simulink model "orion_casestudy_8"  (R2023a)
settings: Solver=VariableStepAuto  StartTime=0.0  StopTime=30  RelTol=1e-3
InitFcn:
  | RandStream.setGlobalStream(RandStream('mt19937ar','seed',sum(100*clock)));
undefined symbols (not defined in the file or in its folder): m, n
(part 2 of 3)

== stateflow chart orion_casestudy_8/Slave3 ==
  settings: updateMethod=CONTINUOUS
  state Connected
    entry:
    connStatus=2;
    state KeepAliveSendTimeout [parallel]
      settings: executionOrder=1
      state KeepAliveSend
      (default) -> KeepAliveSend
      KeepAliveSend -> KeepAliveSend [order 1] : after(delay_array(i)*5,msec)
          |  {OrionKeepAliveOut.data=0;
          | send(OrionKeepAliveOut);i = i + 1;}
      KeepAliveSend -> KeepAliveSend [order 2] : SendDataIn
          | {OrionAppDataOut.data=0;
          | send(OrionAppDataOut);}
    state KeepAliveRecieveTimeout [parallel]
      settings: executionOrder=2
      state KeepAlineRec
      (default) -> KeepAlineRec
      KeepAlineRec -> KeepAlineRec [order 2] : OrionKeepAliveIn
      KeepAlineRec -> KeepAlineRec [order 3] : OrionAppDataIn
  state Closed
    entry:
    connStatus=0;
  state Connecting
    entry:
    connStatus=1;
  Connected -> (junction 6) [order 2] : OrionConnRespIn
  Connected -> (junction 6) [order 3] : OrionConnReqIn
  (default) -> Closed : {i=1;}
  (junction 6) -> Closed
  Connected -> (junction 6) [order 1] : OrionConnConfIn
  KeepAlineRec -> Closed [order 1] : after(delay_array(i)*5,msec)
      | {i = i + 1;}
  Connecting -> (junction 36) [order 6] : OrionAppDataIn
  Connecting -> (junction 36) [order 5] : OrionConnReqIn
  (junction 36) -> Closed
  Connecting -> (junction 36) [order 4] : OrionConnRespIn
  Connecting -> (junction 36) [order 3] : OrionKeepAliveIn
  Closed -> Connecting : OrionConnReqIn
      | {OrionConnRespOut.data=0;
      | send(OrionConnRespOut);}
  Connecting -> Closed [order 1] : after(delay_array(i)*5,msec)
      | {i = i + 1;}
  Connecting -> Connected [order 2] : OrionConnConfIn{OrionConnConfOut.data=0;send(OrionConnConfOut);}
  data: OrionKeepAliveIn input; OrionConnConfOut output; OrionConnRespOut output; OrionKeepAliveOut output; OrionAppDataOut output; OrionAppDataIn input; OrionConnRespIn input; OrionConnReqIn input; OrionConnReqOut output size=1; connStatus output; SendDataIn local; OrionConnConfIn input; delay_array input; i local

== stateflow chart orion_casestudy_8/DelaySwitch41 ==
  state Operation
  state Sending
  (default) -> Operation : {i=0;}
  (junction 7) -> Operation [order 2]
  Sending -> Operation : after(delay_array(i),msec)
      | {receive(inMsg);outMsg.data=0;send(outMsg);}
  Operation -> (junction 7) : inMsg{i = i + 1;}
  (junction 7) -> Sending [order 1] : [switch_array(i)==0]
  data: switch_array input; delay_array input; outMsg output; inMsg input; i local

== stateflow chart orion_casestudy_8/DelaySwitch42 ==
  state Operation
  state Sending
  (default) -> Operation : {i=0;}
  (junction 7) -> Operation [order 2]
  Sending -> Operation : after(delay_array(i),msec)
      | {receive(inMsg);outMsg.data=0;send(outMsg);}
  Operation -> (junction 7) : inMsg{i = i + 1;}
  (junction 7) -> Sending [order 1] : [switch_array(i)==0]
  data: switch_array input; delay_array input; outMsg output; inMsg input; i local

== stateflow chart orion_casestudy_8/DelaySwitch43 ==
  state Operation
  state Sending
  (default) -> Operation : {i=0;}
  (junction 7) -> Operation [order 2]
  Sending -> Operation : after(delay_array(i),msec)
      | {receive(inMsg);outMsg.data=0;send(outMsg);}
  Operation -> (junction 7) : inMsg{i = i + 1;}
  (junction 7) -> Sending [order 1] : [switch_array(i)==0]
  data: switch_array input; delay_array input; outMsg output; inMsg input; i local

== stateflow chart orion_casestudy_8/DelaySwitch44 ==
  state Operation
  state Sending
  (default) -> Operation : {i=0;}
  (junction 7) -> Operation [order 2]
  Sending -> Operation : after(delay_array(i),msec)
      | {receive(inMsg);outMsg.data=0;send(outMsg);}
  Operation -> (junction 7) : inMsg{i = i + 1;}
  (junction 7) -> Sending [order 1] : [switch_array(i)==0]
  data: switch_array input; delay_array input; outMsg output; inMsg input; i local

== stateflow chart orion_casestudy_8/DelaySwitch45 ==
  state Operation
  state Sending
  (default) -> Operation : {i=0;}
  (junction 7) -> Operation [order 2]
  Sending -> Operation : after(delay_array(i),msec)
      | {receive(inMsg);outMsg.data=0;send(outMsg);}
  Operation -> (junction 7) : inMsg{i = i + 1;}
  (junction 7) -> Sending [order 1] : [switch_array(i)==0]
  data: switch_array input; delay_array input; outMsg output; inMsg input; i local

== stateflow chart orion_casestudy_8/DelaySwitch46 ==
  state Operation
  state Sending
  (default) -> Operation : {i=0;}
  (junction 7) -> Operation [order 2]
  Sending -> Operation : after(delay_array(i),msec)
      | {receive(inMsg);outMsg.data=0;send(outMsg);}
  Operation -> (junction 7) : inMsg{i = i + 1;}
  (junction 7) -> Sending [order 1] : [switch_array(i)==0]
  data: switch_array input; delay_array input; outMsg output; inMsg input; i local

== stateflow chart orion_casestudy_8/DelaySwitch47 ==
  state Operation
  state Sending
  (default) -> Operation : {i=0;}
  (junction 7) -> Operation [order 2]
  Sending -> Operation : after(delay_array(i),msec)
      | {receive(inMsg);outMsg.data=0;send(outMsg);}
  Operation -> (junction 7) : inMsg{i = i + 1;}
  (junction 7) -> Sending [order 1] : [switch_array(i)==0]
  data: switch_array input; delay_array input; outMsg output; inMsg input; i local

== stateflow chart orion_casestudy_8/DelaySwitch48 ==
  state Operation
  state Sending
  (default) -> Operation : {i=0;}
  (junction 7) -> Operation [order 2]
  Sending -> Operation : after(delay_array(i),msec)
      | {receive(inMsg);outMsg.data=0;send(outMsg);}
  Operation -> (junction 7) : inMsg{i = i + 1;}
  (junction 7) -> Sending [order 1] : [switch_array(i)==0]
  data: switch_array input; delay_array input; outMsg output; inMsg input; i local

== stateflow chart orion_casestudy_8/DelaySwitch49 ==
  state Operation
  state Sending
  (default) -> Operation : {i=0;}
  (junction 7) -> Operation [order 2]
  Sending -> Operation : after(delay_array(i),msec)
      | {receive(inMsg);outMsg.data=0;send(outMsg);}
  Operation -> (junction 7) : inMsg{i = i + 1;}
  (junction 7) -> Sending [order 1] : [switch_array(i)==0]
  data: switch_array input; delay_array input; outMsg output; inMsg input; i local

== stateflow chart orion_casestudy_8/DelaySwitch50 ==
  state Operation
  state Sending
  (default) -> Operation : {i=0;}
  (junction 7) -> Operation [order 2]
  Sending -> Operation : after(delay_array(i),msec)
      | {receive(inMsg);outMsg.data=0;send(outMsg);}
  Operation -> (junction 7) : inMsg{i = i + 1;}
  (junction 7) -> Sending [order 1] : [switch_array(i)==0]
  data: switch_array input; delay_array input; outMsg output; inMsg input; i local

== stateflow chart orion_casestudy_8/DelaySwitch51 ==
  state Operation
  state Sending
  (default) -> Operation : {i=0;}
  (junction 7) -> Operation [order 2]
  Sending -> Operation : after(delay_array(i),msec)
      | {receive(inMsg);outMsg.data=0;send(outMsg);}
  Operation -> (junction 7) : inMsg{i = i + 1;}
  (junction 7) -> Sending [order 1] : [switch_array(i)==0]
  data: switch_array input; delay_array input; outMsg output; inMsg input; i local

== stateflow chart orion_casestudy_8/DelaySwitch52 ==
  state Operation
  state Sending
  (default) -> Operation : {i=0;}
  (junction 7) -> Operation [order 2]
  Sending -> Operation : after(delay_array(i),msec)
      | {receive(inMsg);outMsg.data=0;send(outMsg);}
  Operation -> (junction 7) : inMsg{i = i + 1;}
  (junction 7) -> Sending [order 1] : [switch_array(i)==0]
  data: switch_array input; delay_array input; outMsg output; inMsg input; i local

== stateflow chart orion_casestudy_8/DelaySwitch53 ==
  state Operation
  state Sending
  (default) -> Operation : {i=0;}
  (junction 7) -> Operation [order 2]
  Sending -> Operation : after(delay_array(i),msec)
      | {receive(inMsg);outMsg.data=0;send(outMsg);}
  Operation -> (junction 7) : inMsg{i = i + 1;}
  (junction 7) -> Sending [order 1] : [switch_array(i)==0]
  data: switch_array input; delay_array input; outMsg output; inMsg input; i local

== stateflow chart orion_casestudy_8/DelaySwitch54 ==
  state Operation
  state Sending
  (default) -> Operation : {i=0;}
  (junction 7) -> Operation [order 2]
  Sending -> Operation : after(delay_array(i),msec)
      | {receive(inMsg);outMsg.data=0;send(outMsg);}
  Operation -> (junction 7) : inMsg{i = i + 1;}
  (junction 7) -> Sending [order 1] : [switch_array(i)==0]
  data: switch_array input; delay_array input; outMsg output; inMsg input; i local

== stateflow chart orion_casestudy_8/DelaySwitch55 ==
  state Operation
  state Sending
  (default) -> Operation : {i=0;}
  (junction 7) -> Operation [order 2]
  Sending -> Operation : after(delay_array(i),msec)
      | {receive(inMsg);outMsg.data=0;send(outMsg);}
  Operation -> (junction 7) : inMsg{i = i + 1;}
  (junction 7) -> Sending [order 1] : [switch_array(i)==0]
  data: switch_array input; delay_array input; outMsg output; inMsg input; i local

== stateflow chart orion_casestudy_8/DelaySwitch56 ==
  state Operation
  state Sending
  (default) -> Operation : {i=0;}
  (junction 7) -> Operation [order 2]
  Sending -> Operation : after(delay_array(i),msec)
      | {receive(inMsg);outMsg.data=0;send(outMsg);}
  Operation -> (junction 7) : inMsg{i = i + 1;}
  (junction 7) -> Sending [order 1] : [switch_array(i)==0]
  data: switch_array input; delay_array input; outMsg output; inMsg input; i local

== stateflow chart orion_casestudy_8/DelaySwitch57 ==
  state Operation
  state Sending
  (default) -> Operation : {i=0;}
  (junction 7) -> Operation [order 2]
  Sending -> Operation : after(delay_array(i),msec)
      | {receive(inMsg);outMsg.data=0;send(outMsg);}
  Operation -> (junction 7) : inMsg{i = i + 1;}
  (junction 7) -> Sending [order 1] : [switch_array(i)==0]
  data: switch_array input; delay_array input; outMsg output; inMsg input; i local

== stateflow chart orion_casestudy_8/DelaySwitch58 ==
  state Operation
  state Sending
  (default) -> Operation : {i=0;}
  (junction 7) -> Operation [order 2]
  Sending -> Operation : after(delay_array(i),msec)
      | {receive(inMsg);outMsg.data=0;send(outMsg);}
  Operation -> (junction 7) : inMsg{i = i + 1;}
  (junction 7) -> Sending [order 1] : [switch_array(i)==0]
  data: switch_array input; delay_array input; outMsg output; inMsg input; i local

== stateflow chart orion_casestudy_8/DelaySwitch59 ==
  state Operation
  state Sending
  (default) -> Operation : {i=0;}
  (junction 7) -> Operation [order 2]
  Sending -> Operation : after(delay_array(i),msec)
      | {receive(inMsg);outMsg.data=0;send(outMsg);}
  Operation -> (junction 7) : inMsg{i = i + 1;}
  (junction 7) -> Sending [order 1] : [switch_array(i)==0]
  data: switch_array input; delay_array input; outMsg output; inMsg input; i local

== stateflow chart orion_casestudy_8/DelaySwitch60 ==
  state Operation
  state Sending
  (default) -> Operation : {i=0;}
  (junction 7) -> Operation [order 2]
  Sending -> Operation : after(delay_array(i),msec)
      | {receive(inMsg);outMsg.data=0;send(outMsg);}
  Operation -> (junction 7) : inMsg{i = i + 1;}
  (junction 7) -> Sending [order 1] : [switch_array(i)==0]
  data: switch_array input; delay_array input; outMsg output; inMsg input; i local

== stateflow chart orion_casestudy_8/DelaySwitch61 ==
  state Operation
  state Sending
  (default) -> Operation : {i=0;}
  (junction 7) -> Operation [order 2]
  Sending -> Operation : after(delay_array(i),msec)
      | {receive(inMsg);outMsg.data=0;send(outMsg);}
  Operation -> (junction 7) : inMsg{i = i + 1;}
  (junction 7) -> Sending [order 1] : [switch_array(i)==0]
  data: switch_array input; delay_array input; outMsg output; inMsg input; i local

== stateflow chart orion_casestudy_8/DelaySwitch62 ==
  state Operation
  state Sending
  (default) -> Operation : {i=0;}
  (junction 7) -> Operation [order 2]
  Sending -> Operation : after(delay_array(i),msec)
      | {receive(inMsg);outMsg.data=0;send(outMsg);}
  Operation -> (junction 7) : inMsg{i = i + 1;}
  (junction 7) -> Sending [order 1] : [switch_array(i)==0]
  data: switch_array input; delay_array input; outMsg output; inMsg input; i local

== stateflow chart orion_casestudy_8/DelaySwitch63 ==
  state Operation
  state Sending
  (default) -> Operation : {i=0;}
  (junction 7) -> Operation [order 2]
  Sending -> Operation : after(delay_array(i),msec)
      | {receive(inMsg);outMsg.data=0;send(outMsg);}
  Operation -> (junction 7) : inMsg{i = i + 1;}
  (junction 7) -> Sending [order 1] : [switch_array(i)==0]
  data: switch_array input; delay_array input; outMsg output; inMsg input; i local

== stateflow chart orion_casestudy_8/DelaySwitch3 ==
  state Operation
  state Sending
  (default) -> Operation : {i=0;}
  (junction 7) -> Operation [order 2]
  Sending -> Operation : after(delay_array(i),msec)
      | {receive(inMsg);outMsg.data=0;send(outMsg);}
  Operation -> (junction 7) : inMsg{i = i + 1;}
  (junction 7) -> Sending [order 1] : [switch_array(i)==0]
  data: switch_array input; delay_array input; outMsg output; inMsg input; i local

== stateflow chart orion_casestudy_8/DelaySwitch64 ==
  state Operation
  state Sending
  (default) -> Operation : {i=0;}
  (junction 7) -> Operation [order 2]
  Sending -> Operation : after(delay_array(i),msec)
      | {receive(inMsg);outMsg.data=0;send(outMsg);}
  Operation -> (junction 7) : inMsg{i = i + 1;}
  (junction 7) -> Sending [order 1] : [switch_array(i)==0]
  data: switch_array input; delay_array input; outMsg output; inMsg input; i local

== stateflow chart orion_casestudy_8/DelaySwitch65 ==
  state Operation
  state Sending
  (default) -> Operation : {i=0;}
  (junction 7) -> Operation [order 2]
  Sending -> Operation : after(delay_array(i),msec)
      | {receive(inMsg);outMsg.data=0;send(outMsg);}
  Operation -> (junction 7) : inMsg{i = i + 1;}
  (junction 7) -> Sending [order 1] : [switch_array(i)==0]
  data: switch_array input; delay_array input; outMsg output; inMsg input; i local

== stateflow chart orion_casestudy_8/DelaySwitch66 ==
  state Operation
  state Sending
  (default) -> Operation : {i=0;}
  (junction 7) -> Operation [order 2]
  Sending -> Operation : after(delay_array(i),msec)
      | {receive(inMsg);outMsg.data=0;send(outMsg);}
  Operation -> (junction 7) : inMsg{i = i + 1;}
  (junction 7) -> Sending [order 1] : [switch_array(i)==0]
  data: switch_array input; delay_array input; outMsg output; inMsg input; i local

== stateflow chart orion_casestudy_8/DelaySwitch67 ==
  state Operation
  state Sending
  (default) -> Operation : {i=0;}
  (junction 7) -> Operation [order 2]
  Sending -> Operation : after(delay_array(i),msec)
      | {receive(inMsg);outMsg.data=0;send(outMsg);}
  Operation -> (junction 7) : inMsg{i = i + 1;}
  (junction 7) -> Sending [order 1] : [switch_array(i)==0]
  data: switch_array input; delay_array input; outMsg output; inMsg input; i local

== stateflow chart orion_casestudy_8/DelaySwitch68 ==
  state Operation
  state Sending
  (default) -> Operation : {i=0;}
  (junction 7) -> Operation [order 2]
  Sending -> Operation : after(delay_array(i),msec)
      | {receive(inMsg);outMsg.data=0;send(outMsg);}
  Operation -> (junction 7) : inMsg{i = i + 1;}
  (junction 7) -> Sending [order 1] : [switch_array(i)==0]
  data: switch_array input; delay_array input; outMsg output; inMsg input; i local

== stateflow chart orion_casestudy_8/DelaySwitch69 ==
  state Operation
  state Sending
  (default) -> Operation : {i=0;}
  (junction 7) -> Operation [order 2]
  Sending -> Operation : after(delay_array(i),msec)
      | {receive(inMsg);outMsg.data=0;send(outMsg);}
  Operation -> (junction 7) : inMsg{i = i + 1;}
  (junction 7) -> Sending [order 1] : [switch_array(i)==0]
  data: switch_array input; delay_array input; outMsg output; inMsg input; i local

== stateflow chart orion_casestudy_8/DelaySwitch70 ==
  state Operation
  state Sending
  (default) -> Operation : {i=0;}
  (junction 7) -> Operation [order 2]
  Sending -> Operation : after(delay_array(i),msec)
      | {receive(inMsg);outMsg.data=0;send(outMsg);}
  Operation -> (junction 7) : inMsg{i = i + 1;}
  (junction 7) -> Sending [order 1] : [switch_array(i)==0]
  data: switch_array input; delay_array input; outMsg output; inMsg input; i local

== stateflow chart orion_casestudy_8/DelaySwitch71 ==
  state Operation
  state Sending
  (default) -> Operation : {i=0;}
  (junction 7) -> Operation [order 2]
  Sending -> Operation : after(delay_array(i),msec)
      | {receive(inMsg);outMsg.data=0;send(outMsg);}
  Operation -> (junction 7) : inMsg{i = i + 1;}
  (junction 7) -> Sending [order 1] : [switch_array(i)==0]
  data: switch_array input; delay_array input; outMsg output; inMsg input; i local

== stateflow chart orion_casestudy_8/DelaySwitch72 ==
  state Operation
  state Sending
  (default) -> Operation : {i=0;}
  (junction 7) -> Operation [order 2]
  Sending -> Operation : after(delay_array(i),msec)
      | {receive(inMsg);outMsg.data=0;send(outMsg);}
  Operation -> (junction 7) : inMsg{i = i + 1;}
  (junction 7) -> Sending [order 1] : [switch_array(i)==0]
  data: switch_array input; delay_array input; outMsg output; inMsg input; i local

== stateflow chart orion_casestudy_8/DelaySwitch73 ==
  state Operation
  state Sending
  (default) -> Operation : {i=0;}
  (junction 7) -> Operation [order 2]
  Sending -> Operation : after(delay_array(i),msec)
      | {receive(inMsg);outMsg.data=0;send(outMsg);}
  Operation -> (junction 7) : inMsg{i = i + 1;}
  (junction 7) -> Sending [order 1] : [switch_array(i)==0]
  data: switch_array input; delay_array input; outMsg output; inMsg input; i local

== stateflow chart orion_casestudy_8/DelaySwitch4 ==
  state Operation
  state Sending
  (default) -> Operation : {i=0;}
  (junction 7) -> Operation [order 2]
  Sending -> Operation : after(delay_array(i),msec)
      | {receive(inMsg);outMsg.data=0;send(outMsg);}
  Operation -> (junction 7) : inMsg{i = i + 1;}
  (junction 7) -> Sending [order 1] : [switch_array(i)==0]
  data: switch_array input; delay_array input; outMsg output; inMsg input; i local

== stateflow chart orion_casestudy_8/DelaySwitch74 ==
  state Operation
  state Sending
  (default) -> Operation : {i=0;}
  (junction 7) -> Operation [order 2]
  Sending -> Operation : after(delay_array(i),msec)
      | {receive(inMsg);outMsg.data=0;send(outMsg);}
  Operation -> (junction 7) : inMsg{i = i + 1;}
  (junction 7) -> Sending [order 1] : [switch_array(i)==0]
  data: switch_array input; delay_array input; outMsg output; inMsg input; i local

== stateflow chart orion_casestudy_8/DelaySwitch75 ==
  state Operation
  state Sending
  (default) -> Operation : {i=0;}
  (junction 7) -> Operation [order 2]
  Sending -> Operation : after(delay_array(i),msec)
      | {receive(inMsg);outMsg.data=0;send(outMsg);}
  Operation -> (junction 7) : inMsg{i = i + 1;}
  (junction 7) -> Sending [order 1] : [switch_array(i)==0]
  data: switch_array input; delay_array input; outMsg output; inMsg input; i local

== stateflow chart orion_casestudy_8/DelaySwitch76 ==
  state Operation
  state Sending
  (default) -> Operation : {i=0;}
  (junction 7) -> Operation [order 2]
  Sending -> Operation : after(delay_array(i),msec)
      | {receive(inMsg);outMsg.data=0;send(outMsg);}
  Operation -> (junction 7) : inMsg{i = i + 1;}
  (junction 7) -> Sending [order 1] : [switch_array(i)==0]
  data: switch_array input; delay_array input; outMsg output; inMsg input; i local

== stateflow chart orion_casestudy_8/DelaySwitch77 ==
  state Operation
  state Sending
  (default) -> Operation : {i=0;}
  (junction 7) -> Operation [order 2]
  Sending -> Operation : after(delay_array(i),msec)
      | {receive(inMsg);outMsg.data=0;send(outMsg);}
  Operation -> (junction 7) : inMsg{i = i + 1;}
  (junction 7) -> Sending [order 1] : [switch_array(i)==0]
  data: switch_array input; delay_array input; outMsg output; inMsg input; i local

== stateflow chart orion_casestudy_8/DelaySwitch78 ==
  state Operation
  state Sending
  (default) -> Operation : {i=0;}
  (junction 7) -> Operation [order 2]
  Sending -> Operation : after(delay_array(i),msec)
      | {receive(inMsg);outMsg.data=0;send(outMsg);}
  Operation -> (junction 7) : inMsg{i = i + 1;}
  (junction 7) -> Sending [order 1] : [switch_array(i)==0]
  data: switch_array input; delay_array input; outMsg output; inMsg input; i local

== stateflow chart orion_casestudy_8/DelaySwitch79 ==
  state Operation
  state Sending
  (default) -> Operation : {i=0;}
  (junction 7) -> Operation [order 2]
  Sending -> Operation : after(delay_array(i),msec)
      | {receive(inMsg);outMsg.data=0;send(outMsg);}
  Operation -> (junction 7) : inMsg{i = i + 1;}
  (junction 7) -> Sending [order 1] : [switch_array(i)==0]
  data: switch_array input; delay_array input; outMsg output; inMsg input; i local

== stateflow chart orion_casestudy_8/DelaySwitch80 ==
  state Operation
  state Sending
  (default) -> Operation : {i=0;}
  (junction 7) -> Operation [order 2]
  Sending -> Operation : after(delay_array(i),msec)
      | {receive(inMsg);outMsg.data=0;send(outMsg);}
  Operation -> (junction 7) : inMsg{i = i + 1;}
  (junction 7) -> Sending [order 1] : [switch_array(i)==0]
  data: switch_array input; delay_array input; outMsg output; inMsg input; i local

== stateflow chart orion_casestudy_8/Master4 ==
  settings: updateMethod=CONTINUOUS
  state Connected
    entry:
    connStatus=2;
    state KeepAliveSendTimeout [parallel]
      settings: executionOrder=1
      state KeepAliveSend
      (default) -> KeepAliveSend
      KeepAliveSend -> KeepAliveSend [order 1] : after(delay_array(i)*5,msec)
          | {OrionKeepAliveOut.data=0;
          | send(OrionKeepAliveOut);
          | i = i + 1;}
      KeepAliveSend -> KeepAliveSend [order 2] : SendDataIn
          | {OrionAppDataOut.data=0;
          | send(OrionAppDataOut);}
    state KeepAliveRecieveTimeout [parallel]
      settings: executionOrder=2
      state KeepAlineRec
      (default) -> KeepAlineRec
      KeepAlineRec -> KeepAlineRec [order 2] : OrionKeepAliveIn
      KeepAlineRec -> KeepAlineRec [order 3] : OrionAppDataIn
  state Closed
    entry:
    connStatus=0;
  state Connecting
    entry:
    connStatus=1;
  Connected -> (junction 6) [order 1] : OrionConnConfIn
  (default) -> Closed : {i=1;}
  Connected -> (junction 6) [order 2] : OrionConnRespIn
  Connected -> (junction 6) [order 3] : OrionConnReqIn
  (junction 6) -> Closed
  KeepAlineRec -> Closed [order 1] : after(delay_array(i)*5,msec)
      | {i = i + 1;}
  Connecting -> (junction 36) [order 5] : OrionConnReqIn
  (junction 36) -> Closed
  Connecting -> (junction 36) [order 4] : OrionConnRespIn
  Connecting -> (junction 36) [order 2] : OrionKeepAliveIn
  Connecting -> Closed [order 3] : after(delay_array(i)*5,msec)
      | {i = i + 1;}
  Closed -> Connecting [order 2] : after(delay_array(i)*5,msec)
      | {OrionConnReqOut.data=0;send(OrionConnReqOut);i = i + 1;}
  Closed -> Connecting [order 1] : OrionConnReqIn
      | {OrionConnRespOut.data=0;send(OrionConnRespOut);}
  Connecting -> Connected [order 1] : OrionConnRespIn
      | {OrionConnConfOut.data=0;
      | send(OrionConnConfOut);}
  data: delay_array input; OrionKeepAliveOut output; OrionKeepAliveIn input; OrionConnConfOut output; OrionConnConfIn input; OrionConnRespOut output; OrionAppDataOut output; OrionAppDataIn input; OrionConnRespIn input; OrionConnReqIn input; OrionConnReqOut output; connStatus output; SendDataIn local; i local

== stateflow chart orion_casestudy_8/DelaySwitch5 ==
  state Operation
  state Sending
  (default) -> Operation : {i=0;}
  (junction 7) -> Operation [order 2]
  Sending -> Operation : after(delay_array(i),msec)
      | {receive(inMsg);outMsg.data=0;send(outMsg);}
  Operation -> (junction 7) : inMsg{i = i + 1;}
  (junction 7) -> Sending [order 1] : [switch_array(i)==0]
  data: switch_array input; delay_array input; outMsg output; inMsg input; i local

== stateflow chart orion_casestudy_8/Master5 ==
  settings: updateMethod=CONTINUOUS
  state Connected
    entry:
    connStatus=2;
    state KeepAliveSendTimeout [parallel]
      settings: executionOrder=1
      state KeepAliveSend
      (default) -> KeepAliveSend
      KeepAliveSend -> KeepAliveSend [order 1] : after(delay_array(i)*5,msec)
          | {OrionKeepAliveOut.data=0;
          | send(OrionKeepAliveOut);
          | i = i + 1;}
      KeepAliveSend -> KeepAliveSend [order 2] : SendDataIn
          | {OrionAppDataOut.data=0;
          | send(OrionAppDataOut);}
    state KeepAliveRecieveTimeout [parallel]
      settings: executionOrder=2
      state KeepAlineRec
      (default) -> KeepAlineRec
      KeepAlineRec -> KeepAlineRec [order 2] : OrionKeepAliveIn
      KeepAlineRec -> KeepAlineRec [order 3] : OrionAppDataIn
  state Closed
    entry:
    connStatus=0;
  state Connecting
    entry:
    connStatus=1;
  Connected -> (junction 6) [order 1] : OrionConnConfIn
  (default) -> Closed : {i=1;}
  Connected -> (junction 6) [order 2] : OrionConnRespIn
  Connected -> (junction 6) [order 3] : OrionConnReqIn
  (junction 6) -> Closed
  KeepAlineRec -> Closed [order 1] : after(delay_array(i)*5,msec)
      | {i = i + 1;}
  Connecting -> (junction 36) [order 5] : OrionConnReqIn
  (junction 36) -> Closed
  Connecting -> (junction 36) [order 4] : OrionConnRespIn
  Connecting -> (junction 36) [order 2] : OrionKeepAliveIn
  Connecting -> Closed [order 3] : after(delay_array(i)*5,msec)
      | {i = i + 1;}
  Closed -> Connecting [order 2] : after(delay_array(i)*5,msec)
      | {OrionConnReqOut.data=0;send(OrionConnReqOut);i = i + 1;}
  Closed -> Connecting [order 1] : OrionConnReqIn
      | {OrionConnRespOut.data=0;send(OrionConnRespOut);}
  Connecting -> Connected [order 1] : OrionConnRespIn
      | {OrionConnConfOut.data=0;
      | send(OrionConnConfOut);}
  data: delay_array input; OrionKeepAliveOut output; OrionKeepAliveIn input; OrionConnConfOut output; OrionConnConfIn input; OrionConnRespOut output; OrionAppDataOut output; OrionAppDataIn input; OrionConnRespIn input; OrionConnReqIn input; OrionConnReqOut output; connStatus output; SendDataIn local; i local

== stateflow chart orion_casestudy_8/Master6 ==
  settings: updateMethod=CONTINUOUS
  state Connected
    entry:
    connStatus=2;
    state KeepAliveSendTimeout [parallel]
      settings: executionOrder=1
      state KeepAliveSend
      (default) -> KeepAliveSend
      KeepAliveSend -> KeepAliveSend [order 1] : after(delay_array(i)*5,msec)
          | {OrionKeepAliveOut.data=0;
          | send(OrionKeepAliveOut);
          | i = i + 1;}
      KeepAliveSend -> KeepAliveSend [order 2] : SendDataIn
          | {OrionAppDataOut.data=0;
          | send(OrionAppDataOut);}
    state KeepAliveRecieveTimeout [parallel]
      settings: executionOrder=2
      state KeepAlineRec
      (default) -> KeepAlineRec
      KeepAlineRec -> KeepAlineRec [order 2] : OrionKeepAliveIn
      KeepAlineRec -> KeepAlineRec [order 3] : OrionAppDataIn
  state Closed
    entry:
    connStatus=0;
  state Connecting
    entry:
    connStatus=1;
  Connected -> (junction 6) [order 1] : OrionConnConfIn
  (default) -> Closed : {i=1;}
  Connected -> (junction 6) [order 2] : OrionConnRespIn
  Connected -> (junction 6) [order 3] : OrionConnReqIn
  (junction 6) -> Closed
  KeepAlineRec -> Closed [order 1] : after(delay_array(i)*5,msec)
      | {i = i + 1;}
  Connecting -> (junction 36) [order 5] : OrionConnReqIn
  (junction 36) -> Closed
  Connecting -> (junction 36) [order 4] : OrionConnRespIn
  Connecting -> (junction 36) [order 2] : OrionKeepAliveIn
  Connecting -> Closed [order 3] : after(delay_array(i)*5,msec)
      | {i = i + 1;}
  Closed -> Connecting [order 2] : after(delay_array(i)*5,msec)
      | {OrionConnReqOut.data=0;send(OrionConnReqOut);i = i + 1;}
  Closed -> Connecting [order 1] : OrionConnReqIn
      | {OrionConnRespOut.data=0;send(OrionConnRespOut);}
  Connecting -> Connected [order 1] : OrionConnRespIn
      | {OrionConnConfOut.data=0;
      | send(OrionConnConfOut);}
  data: delay_array input; OrionKeepAliveOut output; OrionKeepAliveIn input; OrionConnConfOut output; OrionConnConfIn input; OrionConnRespOut output; OrionAppDataOut output; OrionAppDataIn input; OrionConnRespIn input; OrionConnReqIn input; OrionConnReqOut output; connStatus output; SendDataIn local; i local

== stateflow chart orion_casestudy_8/Master7 ==
  settings: updateMethod=CONTINUOUS
  state Connected
    entry:
    connStatus=2;
    state KeepAliveSendTimeout [parallel]
      settings: executionOrder=1
      state KeepAliveSend
      (default) -> KeepAliveSend
      KeepAliveSend -> KeepAliveSend [order 1] : after(delay_array(i)*5,msec)
          | {OrionKeepAliveOut.data=0;
          | send(OrionKeepAliveOut);
          | i = i + 1;}
      KeepAliveSend -> KeepAliveSend [order 2] : SendDataIn
          | {OrionAppDataOut.data=0;
          | send(OrionAppDataOut);}
    state KeepAliveRecieveTimeout [parallel]
      settings: executionOrder=2
      state KeepAlineRec
      (default) -> KeepAlineRec
      KeepAlineRec -> KeepAlineRec [order 2] : OrionKeepAliveIn
      KeepAlineRec -> KeepAlineRec [order 3] : OrionAppDataIn
  state Closed
    entry:
    connStatus=0;
  state Connecting
    entry:
    connStatus=1;
  Connected -> (junction 6) [order 1] : OrionConnConfIn
  (default) -> Closed : {i=1;}
  Connected -> (junction 6) [order 2] : OrionConnRespIn
  Connected -> (junction 6) [order 3] : OrionConnReqIn
  (junction 6) -> Closed
  KeepAlineRec -> Closed [order 1] : after(delay_array(i)*5,msec)
      | {i = i + 1;}
  Connecting -> (junction 36) [order 5] : OrionConnReqIn
  (junction 36) -> Closed
  Connecting -> (junction 36) [order 4] : OrionConnRespIn
  Connecting -> (junction 36) [order 2] : OrionKeepAliveIn
  Connecting -> Closed [order 3] : after(delay_array(i)*5,msec)
      | {i = i + 1;}
  Closed -> Connecting [order 2] : after(delay_array(i)*5,msec)
      | {OrionConnReqOut.data=0;send(OrionConnReqOut);i = i + 1;}
  Closed -> Connecting [order 1] : OrionConnReqIn
      | {OrionConnRespOut.data=0;send(OrionConnRespOut);}
  Connecting -> Connected [order 1] : OrionConnRespIn
      | {OrionConnConfOut.data=0;
      | send(OrionConnConfOut);}
  data: delay_array input; OrionKeepAliveOut output; OrionKeepAliveIn input; OrionConnConfOut output; OrionConnConfIn input; OrionConnRespOut output; OrionAppDataOut output; OrionAppDataIn input; OrionConnRespIn input; OrionConnReqIn input; OrionConnReqOut output; connStatus output; SendDataIn local; i local

== stateflow chart orion_casestudy_8/Slave4 ==
  settings: updateMethod=CONTINUOUS
  state Connected
    entry:
    connStatus=2;
    state KeepAliveSendTimeout [parallel]
      settings: executionOrder=1
      state KeepAliveSend
      (default) -> KeepAliveSend
      KeepAliveSend -> KeepAliveSend [order 1] : after(delay_array(i)*5,msec)
          |  {OrionKeepAliveOut.data=0;
          | send(OrionKeepAliveOut);i = i + 1;}
      KeepAliveSend -> KeepAliveSend [order 2] : SendDataIn
          | {OrionAppDataOut.data=0;
          | send(OrionAppDataOut);}
    state KeepAliveRecieveTimeout [parallel]
      settings: executionOrder=2
      state KeepAlineRec
      (default) -> KeepAlineRec
      KeepAlineRec -> KeepAlineRec [order 2] : OrionKeepAliveIn
      KeepAlineRec -> KeepAlineRec [order 3] : OrionAppDataIn
  state Closed
    entry:
    connStatus=0;
  state Connecting
    entry:
    connStatus=1;
  Connected -> (junction 6) [order 2] : OrionConnRespIn
  Connected -> (junction 6) [order 3] : OrionConnReqIn
  (default) -> Closed : {i=1;}
  (junction 6) -> Closed
  Connected -> (junction 6) [order 1] : OrionConnConfIn
  KeepAlineRec -> Closed [order 1] : after(delay_array(i)*5,msec)
      | {i = i + 1;}
  Connecting -> (junction 36) [order 6] : OrionAppDataIn
  Connecting -> (junction 36) [order 5] : OrionConnReqIn
  (junction 36) -> Closed
  Connecting -> (junction 36) [order 4] : OrionConnRespIn
  Connecting -> (junction 36) [order 3] : OrionKeepAliveIn
  Closed -> Connecting : OrionConnReqIn
      | {OrionConnRespOut.data=0;
      | send(OrionConnRespOut);}
  Connecting -> Closed [order 1] : after(delay_array(i)*5,msec)
      | {i = i + 1;}
  Connecting -> Connected [order 2] : OrionConnConfIn{OrionConnConfOut.data=0;send(OrionConnConfOut);}
  data: OrionKeepAliveIn input; OrionConnConfOut output; OrionConnRespOut output; OrionKeepAliveOut output; OrionAppDataOut output; OrionAppDataIn input; OrionConnRespIn input; OrionConnReqIn input; OrionConnReqOut output size=1; connStatus output; SendDataIn local; OrionConnConfIn input; delay_array input; i local

== stateflow chart orion_casestudy_8/DelaySwitch6 ==
  state Operation
  state Sending
  (default) -> Operation : {i=0;}
  (junction 7) -> Operation [order 2]
  Sending -> Operation : after(delay_array(i),msec)
      | {receive(inMsg);outMsg.data=0;send(outMsg);}
  Operation -> (junction 7) : inMsg{i = i + 1;}
  (junction 7) -> Sending [order 1] : [switch_array(i)==0]
  data: switch_array input; delay_array input; outMsg output; inMsg input; i local

== stateflow chart orion_casestudy_8/Slave5 ==
  settings: updateMethod=CONTINUOUS
  state Connected
    entry:
    connStatus=2;
    state KeepAliveSendTimeout [parallel]
      settings: executionOrder=1
      state KeepAliveSend
      (default) -> KeepAliveSend
      KeepAliveSend -> KeepAliveSend [order 1] : after(delay_array(i)*5,msec)
          |  {OrionKeepAliveOut.data=0;
          | send(OrionKeepAliveOut);i = i + 1;}
      KeepAliveSend -> KeepAliveSend [order 2] : SendDataIn
          | {OrionAppDataOut.data=0;
          | send(OrionAppDataOut);}
    state KeepAliveRecieveTimeout [parallel]
      settings: executionOrder=2
      state KeepAlineRec
      (default) -> KeepAlineRec
      KeepAlineRec -> KeepAlineRec [order 2] : OrionKeepAliveIn
      KeepAlineRec -> KeepAlineRec [order 3] : OrionAppDataIn
  state Closed
    entry:
    connStatus=0;
  state Connecting
    entry:
    connStatus=1;
  Connected -> (junction 6) [order 2] : OrionConnRespIn
  Connected -> (junction 6) [order 3] : OrionConnReqIn
  (default) -> Closed : {i=1;}
  (junction 6) -> Closed
  Connected -> (junction 6) [order 1] : OrionConnConfIn
  KeepAlineRec -> Closed [order 1] : after(delay_array(i)*5,msec)
      | {i = i + 1;}
  Connecting -> (junction 36) [order 6] : OrionAppDataIn
  Connecting -> (junction 36) [order 5] : OrionConnReqIn
  (junction 36) -> Closed
  Connecting -> (junction 36) [order 4] : OrionConnRespIn
  Connecting -> (junction 36) [order 3] : OrionKeepAliveIn
  Closed -> Connecting : OrionConnReqIn
      | {OrionConnRespOut.data=0;
      | send(OrionConnRespOut);}
  Connecting -> Closed [order 1] : after(delay_array(i)*5,msec)
      | {i = i + 1;}
  Connecting -> Connected [order 2] : OrionConnConfIn{OrionConnConfOut.data=0;send(OrionConnConfOut);}
  data: OrionKeepAliveIn input; OrionConnConfOut output; OrionConnRespOut output; OrionKeepAliveOut output; OrionAppDataOut output; OrionAppDataIn input; OrionConnRespIn input; OrionConnReqIn input; OrionConnReqOut output size=1; connStatus output; SendDataIn local; OrionConnConfIn input; delay_array input; i local

== stateflow chart orion_casestudy_8/Slave6 ==
  settings: updateMethod=CONTINUOUS
  state Connected
    entry:
    connStatus=2;
    state KeepAliveSendTimeout [parallel]
      settings: executionOrder=1
      state KeepAliveSend
      (default) -> KeepAliveSend
      KeepAliveSend -> KeepAliveSend [order 1] : after(delay_array(i)*5,msec)
          |  {OrionKeepAliveOut.data=0;
          | send(OrionKeepAliveOut);i = i + 1;}
      KeepAliveSend -> KeepAliveSend [order 2] : SendDataIn
          | {OrionAppDataOut.data=0;
          | send(OrionAppDataOut);}
    state KeepAliveRecieveTimeout [parallel]
      settings: executionOrder=2
      state KeepAlineRec
      (default) -> KeepAlineRec
      KeepAlineRec -> KeepAlineRec [order 2] : OrionKeepAliveIn
      KeepAlineRec -> KeepAlineRec [order 3] : OrionAppDataIn
  state Closed
    entry:
    connStatus=0;
  state Connecting
    entry:
    connStatus=1;
  Connected -> (junction 6) [order 2] : OrionConnRespIn
  Connected -> (junction 6) [order 3] : OrionConnReqIn
  (default) -> Closed : {i=1;}
  (junction 6) -> Closed
  Connected -> (junction 6) [order 1] : OrionConnConfIn
  KeepAlineRec -> Closed [order 1] : after(delay_array(i)*5,msec)
      | {i = i + 1;}
  Connecting -> (junction 36) [order 6] : OrionAppDataIn
  Connecting -> (junction 36) [order 5] : OrionConnReqIn
  (junction 36) -> Closed
  Connecting -> (junction 36) [order 4] : OrionConnRespIn
  Connecting -> (junction 36) [order 3] : OrionKeepAliveIn
  Closed -> Connecting : OrionConnReqIn
      | {OrionConnRespOut.data=0;
      | send(OrionConnRespOut);}
  Connecting -> Closed [order 1] : after(delay_array(i)*5,msec)
      | {i = i + 1;}
  Connecting -> Connected [order 2] : OrionConnConfIn{OrionConnConfOut.data=0;send(OrionConnConfOut);}
  data: OrionKeepAliveIn input; OrionConnConfOut output; OrionConnRespOut output; OrionKeepAliveOut output; OrionAppDataOut output; OrionAppDataIn input; OrionConnRespIn input; OrionConnReqIn input; OrionConnReqOut output size=1; connStatus output; SendDataIn local; OrionConnConfIn input; delay_array input; i local

== stateflow chart orion_casestudy_8/Slave7 ==
  settings: updateMethod=CONTINUOUS
  state Connected
    entry:
    connStatus=2;
    state KeepAliveSendTimeout [parallel]
      settings: executionOrder=1
      state KeepAliveSend
      (default) -> KeepAliveSend
      KeepAliveSend -> KeepAliveSend [order 1] : after(delay_array(i)*5,msec)
          |  {OrionKeepAliveOut.data=0;
          | send(OrionKeepAliveOut);i = i + 1;}
      KeepAliveSend -> KeepAliveSend [order 2] : SendDataIn
          | {OrionAppDataOut.data=0;
          | send(OrionAppDataOut);}
    state KeepAliveRecieveTimeout [parallel]
      settings: executionOrder=2
      state KeepAlineRec
      (default) -> KeepAlineRec
      KeepAlineRec -> KeepAlineRec [order 2] : OrionKeepAliveIn
      KeepAlineRec -> KeepAlineRec [order 3] : OrionAppDataIn
  state Closed
    entry:
    connStatus=0;
  state Connecting
    entry:
    connStatus=1;
  Connected -> (junction 6) [order 2] : OrionConnRespIn
  Connected -> (junction 6) [order 3] : OrionConnReqIn
  (default) -> Closed : {i=1;}
  (junction 6) -> Closed
  Connected -> (junction 6) [order 1] : OrionConnConfIn
  KeepAlineRec -> Closed [order 1] : after(delay_array(i)*5,msec)
      | {i = i + 1;}
  Connecting -> (junction 36) [order 6] : OrionAppDataIn
  Connecting -> (junction 36) [order 5] : OrionConnReqIn
  (junction 36) -> Closed
  Connecting -> (junction 36) [order 4] : OrionConnRespIn
  Connecting -> (junction 36) [order 3] : OrionKeepAliveIn
  Closed -> Connecting : OrionConnReqIn
      | {OrionConnRespOut.data=0;
      | send(OrionConnRespOut);}
  Connecting -> Closed [order 1] : after(delay_array(i)*5,msec)
      | {i = i + 1;}
  Connecting -> Connected [order 2] : OrionConnConfIn{OrionConnConfOut.data=0;send(OrionConnConfOut);}
  data: OrionKeepAliveIn input; OrionConnConfOut output; OrionConnRespOut output; OrionKeepAliveOut output; OrionAppDataOut output; OrionAppDataIn input; OrionConnRespIn input; OrionConnReqIn input; OrionConnReqOut output size=1; connStatus output; SendDataIn local; OrionConnConfIn input; delay_array input; i local

== stateflow chart orion_casestudy_8/Slave ==
  settings: updateMethod=CONTINUOUS
  state Connected
    entry:
    connStatus=2;
    state KeepAliveSendTimeout [parallel]
      settings: executionOrder=1
      state KeepAliveSend
      (default) -> KeepAliveSend
      KeepAliveSend -> KeepAliveSend [order 1] : after(delay_array(i)*5,msec)
          |  {OrionKeepAliveOut.data=0;
          | send(OrionKeepAliveOut);i = i + 1;}
      KeepAliveSend -> KeepAliveSend [order 2] : SendDataIn
          | {OrionAppDataOut.data=0;
          | send(OrionAppDataOut);}
    state KeepAliveRecieveTimeout [parallel]
      settings: executionOrder=2
      state KeepAlineRec
      (default) -> KeepAlineRec
      KeepAlineRec -> KeepAlineRec [order 2] : OrionKeepAliveIn
      KeepAlineRec -> KeepAlineRec [order 3] : OrionAppDataIn
  state Closed
    entry:
    connStatus=0;
  state Connecting
    entry:
    connStatus=1;
  Connected -> (junction 6) [order 2] : OrionConnRespIn
  Connected -> (junction 6) [order 3] : OrionConnReqIn
  (default) -> Closed : {i=1;}
  (junction 6) -> Closed
  Connected -> (junction 6) [order 1] : OrionConnConfIn
  KeepAlineRec -> Closed [order 1] : after(delay_array(i)*5,msec)
      | {i = i + 1;}
  Connecting -> (junction 36) [order 6] : OrionAppDataIn
  Connecting -> (junction 36) [order 5] : OrionConnReqIn
  (junction 36) -> Closed
  Connecting -> (junction 36) [order 4] : OrionConnRespIn
  Connecting -> (junction 36) [order 3] : OrionKeepAliveIn
  Closed -> Connecting : OrionConnReqIn
      | {OrionConnRespOut.data=0;
      | send(OrionConnRespOut);}
  Connecting -> Closed [order 1] : after(delay_array(i)*5,msec)
      | {i = i + 1;}
  Connecting -> Connected [order 2] : OrionConnConfIn{OrionConnConfOut.data=0;send(OrionConnConfOut);}
  data: OrionKeepAliveIn input; OrionConnConfOut output; OrionConnRespOut output; OrionKeepAliveOut output; OrionAppDataOut output; OrionAppDataIn input; OrionConnRespIn input; OrionConnReqIn input; OrionConnReqOut output size=1; connStatus output; SendDataIn local; OrionConnConfIn input; delay_array input; i local

== stateflow chart orion_casestudy_8/DelaySwitch7 ==
  state Operation
  state Sending
  (default) -> Operation : {i=0;}
  (junction 7) -> Operation [order 2]
  Sending -> Operation : after(delay_array(i),msec)
      | {receive(inMsg);outMsg.data=0;send(outMsg);}
  Operation -> (junction 7) : inMsg{i = i + 1;}
  (junction 7) -> Sending [order 1] : [switch_array(i)==0]
  data: switch_array input; delay_array input; outMsg output; inMsg input; i local

== stateflow chart orion_casestudy_8/DelaySwitch8 ==
  state Operation
  state Sending
  (default) -> Operation : {i=0;}
  (junction 7) -> Operation [order 2]
  Sending -> Operation : after(delay_array(i),msec)
      | {receive(inMsg);outMsg.data=0;send(outMsg);}
  Operation -> (junction 7) : inMsg{i = i + 1;}
  (junction 7) -> Sending [order 1] : [switch_array(i)==0]
  data: switch_array input; delay_array input; outMsg output; inMsg input; i local

== stateflow chart orion_casestudy_8/DelaySwitch9 ==
  state Operation
  state Sending
  (default) -> Operation : {i=0;}
  (junction 7) -> Operation [order 2]
  Sending -> Operation : after(delay_array(i),msec)
      | {receive(inMsg);outMsg.data=0;send(outMsg);}
  Operation -> (junction 7) : inMsg{i = i + 1;}
  (junction 7) -> Sending [order 1] : [switch_array(i)==0]
  data: switch_array input; delay_array input; outMsg output; inMsg input; i local

== stateflow chart orion_casestudy_8/DelaySwitch10 ==
  state Operation
  state Sending
  (default) -> Operation : {i=0;}
  (junction 7) -> Operation [order 2]
  Sending -> Operation : after(delay_array(i),msec)
      | {receive(inMsg);outMsg.data=0;send(outMsg);}
  Operation -> (junction 7) : inMsg{i = i + 1;}
  (junction 7) -> Sending [order 1] : [switch_array(i)==0]
  data: switch_array input; delay_array input; outMsg output; inMsg input; i local

== stateflow chart orion_casestudy_8/OverallState ==
  settings: updateMethod=CONTINUOUS
  state NotConnected
    op_time=temporalCount(msec);
  state Connected
    entry:
    connStatus=1;
  (default) -> NotConnected : {connStatus=0;
      | op_time=0;}
  NotConnected -> Connected : [(conn1==2 && conn2==2) ||  (conn3==2 && conn4==2) ||  (conn5==2 && conn6==2) ||  (conn7==2 && conn8==2) ||  (conn9==2 && conn10==2) ||  (conn11==2 && conn12==2) ||  (conn13==2 && conn14==2) ||  (conn15==2 && conn16==2)]
  data: conn1 input; conn2 input; connStatus output; op_time output; conn3 input; conn4 input; conn5 input; conn6 input; conn7 input; conn8 input; conn9 input; conn10 input; conn11 input; conn12 input; conn13 input; conn14 input; conn15 input; conn16 input

== stateflow chart orion_casestudy_8/DelaySwitch11 ==
  state Operation
  state Sending
  (default) -> Operation : {i=0;}
  (junction 7) -> Operation [order 2]
  Sending -> Operation : after(delay_array(i),msec)
      | {receive(inMsg);outMsg.data=0;send(outMsg);}
  Operation -> (junction 7) : inMsg{i = i + 1;}
  (junction 7) -> Sending [order 1] : [switch_array(i)==0]
  data: switch_array input; delay_array input; outMsg output; inMsg input; i local

== stateflow chart orion_casestudy_8/DelaySwitch12 ==
  state Operation
  state Sending
  (default) -> Operation : {i=0;}
  (junction 7) -> Operation [order 2]
  Sending -> Operation : after(delay_array(i),msec)
      | {receive(inMsg);outMsg.data=0;send(outMsg);}
  Operation -> (junction 7) : inMsg{i = i + 1;}
  (junction 7) -> Sending [order 1] : [switch_array(i)==0]
  data: switch_array input; delay_array input; outMsg output; inMsg input; i local

== stateflow chart orion_casestudy_8/DelaySwitch13 ==
  state Operation
  state Sending
  (default) -> Operation : {i=0;}
  (junction 7) -> Operation [order 2]
  Sending -> Operation : after(delay_array(i),msec)
      | {receive(inMsg);outMsg.data=0;send(outMsg);}
  Operation -> (junction 7) : inMsg{i = i + 1;}
  (junction 7) -> Sending [order 1] : [switch_array(i)==0]
  data: switch_array input; delay_array input; outMsg output; inMsg input; i local

== stateflow chart orion_casestudy_8/DelaySwitch14 ==
  state Operation
  state Sending
  (default) -> Operation : {i=0;}
  (junction 7) -> Operation [order 2]
  Sending -> Operation : after(delay_array(i),msec)
      | {receive(inMsg);outMsg.data=0;send(outMsg);}
  Operation -> (junction 7) : inMsg{i = i + 1;}
  (junction 7) -> Sending [order 1] : [switch_array(i)==0]
  data: switch_array input; delay_array input; outMsg output; inMsg input; i local

== stateflow chart orion_casestudy_8/DelaySwitch15 ==
  state Operation
  state Sending
  (default) -> Operation : {i=0;}
  (junction 7) -> Operation [order 2]
  Sending -> Operation : after(delay_array(i),msec)
      | {receive(inMsg);outMsg.data=0;send(outMsg);}
  Operation -> (junction 7) : inMsg{i = i + 1;}
  (junction 7) -> Sending [order 1] : [switch_array(i)==0]
  data: switch_array input; delay_array input; outMsg output; inMsg input; i local

== stateflow chart orion_casestudy_8/DelaySwitch16 ==
  state Operation
  state Sending
  (default) -> Operation : {i=0;}
  (junction 7) -> Operation [order 2]
  Sending -> Operation : after(delay_array(i),msec)
      | {receive(inMsg);outMsg.data=0;send(outMsg);}
  Operation -> (junction 7) : inMsg{i = i + 1;}
  (junction 7) -> Sending [order 1] : [switch_array(i)==0]
  data: switch_array input; delay_array input; outMsg output; inMsg input; i local

== stateflow chart orion_casestudy_8/DelaySwitch17 ==
  state Operation
  state Sending
  (default) -> Operation : {i=0;}
  (junction 7) -> Operation [order 2]
  Sending -> Operation : after(delay_array(i),msec)
      | {receive(inMsg);outMsg.data=0;send(outMsg);}
  Operation -> (junction 7) : inMsg{i = i + 1;}
  (junction 7) -> Sending [order 1] : [switch_array(i)==0]
  data: switch_array input; delay_array input; outMsg output; inMsg input; i local

== stateflow chart orion_casestudy_8/DelaySwitch18 ==
  state Operation
  state Sending
  (default) -> Operation : {i=0;}
  (junction 7) -> Operation [order 2]
  Sending -> Operation : after(delay_array(i),msec)
      | {receive(inMsg);outMsg.data=0;send(outMsg);}
  Operation -> (junction 7) : inMsg{i = i + 1;}
  (junction 7) -> Sending [order 1] : [switch_array(i)==0]
  data: switch_array input; delay_array input; outMsg output; inMsg input; i local

== stateflow chart orion_casestudy_8/DelaySwitch19 ==
  state Operation
  state Sending
  (default) -> Operation : {i=0;}
  (junction 7) -> Operation [order 2]
  Sending -> Operation : after(delay_array(i),msec)
      | {receive(inMsg);outMsg.data=0;send(outMsg);}
  Operation -> (junction 7) : inMsg{i = i + 1;}
  (junction 7) -> Sending [order 1] : [switch_array(i)==0]
  data: switch_array input; delay_array input; outMsg output; inMsg input; i local

== stateflow chart orion_casestudy_8/DelaySwitch20 ==
  state Operation
  state Sending
  (default) -> Operation : {i=0;}
  (junction 7) -> Operation [order 2]
  Sending -> Operation : after(delay_array(i),msec)
      | {receive(inMsg);outMsg.data=0;send(outMsg);}
  Operation -> (junction 7) : inMsg{i = i + 1;}
  (junction 7) -> Sending [order 1] : [switch_array(i)==0]
  data: switch_array input; delay_array input; outMsg output; inMsg input; i local

== stateflow chart orion_casestudy_8/Master1 ==
  settings: updateMethod=CONTINUOUS
  state Connected
    entry:
    connStatus=2;
    state KeepAliveSendTimeout [parallel]
      settings: executionOrder=1
      state KeepAliveSend
      (default) -> KeepAliveSend
      KeepAliveSend -> KeepAliveSend [order 1] : after(delay_array(i)*5,msec)
          | {OrionKeepAliveOut.data=0;
          | send(OrionKeepAliveOut);
          | i = i + 1;}
      KeepAliveSend -> KeepAliveSend [order 2] : SendDataIn
          | {OrionAppDataOut.data=0;
          | send(OrionAppDataOut);}
    state KeepAliveRecieveTimeout [parallel]
      settings: executionOrder=2
      state KeepAlineRec
      (default) -> KeepAlineRec
      KeepAlineRec -> KeepAlineRec [order 2] : OrionKeepAliveIn
      KeepAlineRec -> KeepAlineRec [order 3] : OrionAppDataIn
  state Closed
    entry:
    connStatus=0;
  state Connecting
    entry:
    connStatus=1;
  Connected -> (junction 6) [order 1] : OrionConnConfIn
  (default) -> Closed : {i=1;}
  Connected -> (junction 6) [order 2] : OrionConnRespIn
  Connected -> (junction 6) [order 3] : OrionConnReqIn
  (junction 6) -> Closed
  KeepAlineRec -> Closed [order 1] : after(delay_array(i)*5,msec)
      | {i = i + 1;}
  Connecting -> (junction 36) [order 5] : OrionConnReqIn
  (junction 36) -> Closed
  Connecting -> (junction 36) [order 4] : OrionConnRespIn
  Connecting -> (junction 36) [order 2] : OrionKeepAliveIn
  Connecting -> Closed [order 3] : after(delay_array(i)*5,msec)
      | {i = i + 1;}
  Closed -> Connecting [order 2] : after(delay_array(i)*5,msec)
      | {OrionConnReqOut.data=0;send(OrionConnReqOut);i = i + 1;}
  Closed -> Connecting [order 1] : OrionConnReqIn
      | {OrionConnRespOut.data=0;send(OrionConnRespOut);}
  Connecting -> Connected [order 1] : OrionConnRespIn
      | {OrionConnConfOut.data=0;
      | send(OrionConnConfOut);}
  data: delay_array input; OrionKeepAliveOut output; OrionKeepAliveIn input; OrionConnConfOut output; OrionConnConfIn input; OrionConnRespOut output; OrionAppDataOut output; OrionAppDataIn input; OrionConnRespIn input; OrionConnReqIn input; OrionConnReqOut output; connStatus output; SendDataIn local; i local

== stateflow chart orion_casestudy_8/Slave1 ==
  settings: updateMethod=CONTINUOUS
  state Connected
    entry:
    connStatus=2;
    state KeepAliveSendTimeout [parallel]
      settings: executionOrder=1
      state KeepAliveSend
      (default) -> KeepAliveSend
      KeepAliveSend -> KeepAliveSend [order 1] : after(delay_array(i)*5,msec)
          |  {OrionKeepAliveOut.data=0;
          | send(OrionKeepAliveOut);i = i + 1;}
      KeepAliveSend -> KeepAliveSend [order 2] : SendDataIn
          | {OrionAppDataOut.data=0;
          | send(OrionAppDataOut);}
    state KeepAliveRecieveTimeout [parallel]
      settings: executionOrder=2
      state KeepAlineRec
      (default) -> KeepAlineRec
      KeepAlineRec -> KeepAlineRec [order 2] : OrionKeepAliveIn
      KeepAlineRec -> KeepAlineRec [order 3] : OrionAppDataIn
  state Closed
    entry:
    connStatus=0;
  state Connecting
    entry:
    connStatus=1;
  Connected -> (junction 6) [order 2] : OrionConnRespIn
  Connected -> (junction 6) [order 3] : OrionConnReqIn
  (default) -> Closed : {i=1;}
  (junction 6) -> Closed
  Connected -> (junction 6) [order 1] : OrionConnConfIn
  KeepAlineRec -> Closed [order 1] : after(delay_array(i)*5,msec)
      | {i = i + 1;}
  Connecting -> (junction 36) [order 6] : OrionAppDataIn
  Connecting -> (junction 36) [order 5] : OrionConnReqIn
  (junction 36) -> Closed
  Connecting -> (junction 36) [order 4] : OrionConnRespIn
  Connecting -> (junction 36) [order 3] : OrionKeepAliveIn
  Closed -> Connecting : OrionConnReqIn
      | {OrionConnRespOut.data=0;
      | send(OrionConnRespOut);}
  Connecting -> Closed [order 1] : after(delay_array(i)*5,msec)
      | {i = i + 1;}
  Connecting -> Connected [order 2] : OrionConnConfIn{OrionConnConfOut.data=0;send(OrionConnConfOut);}
  data: OrionKeepAliveIn input; OrionConnConfOut output; OrionConnRespOut output; OrionKeepAliveOut output; OrionAppDataOut output; OrionAppDataIn input; OrionConnRespIn input; OrionConnReqIn input; OrionConnReqOut output size=1; connStatus output; SendDataIn local; OrionConnConfIn input; delay_array input; i local

== stateflow chart orion_casestudy_8/DelaySwitch21 ==
  state Operation
  state Sending
  (default) -> Operation : {i=0;}
  (junction 7) -> Operation [order 2]
  Sending -> Operation : after(delay_array(i),msec)
      | {receive(inMsg);outMsg.data=0;send(outMsg);}
  Operation -> (junction 7) : inMsg{i = i + 1;}
  (junction 7) -> Sending [order 1] : [switch_array(i)==0]
  data: switch_array input; delay_array input; outMsg output; inMsg input; i local

== stateflow chart orion_casestudy_8/DelaySwitch22 ==
  state Operation
  state Sending
  (default) -> Operation : {i=0;}
  (junction 7) -> Operation [order 2]
  Sending -> Operation : after(delay_array(i),msec)
      | {receive(inMsg);outMsg.data=0;send(outMsg);}
  Operation -> (junction 7) : inMsg{i = i + 1;}
  (junction 7) -> Sending [order 1] : [switch_array(i)==0]
  data: switch_array input; delay_array input; outMsg output; inMsg input; i local

== stateflow chart orion_casestudy_8/DelaySwitch23 ==
  state Operation
  state Sending
  (default) -> Operation : {i=0;}
  (junction 7) -> Operation [order 2]
  Sending -> Operation : after(delay_array(i),msec)
      | {receive(inMsg);outMsg.data=0;send(outMsg);}
  Operation -> (junction 7) : inMsg{i = i + 1;}
  (junction 7) -> Sending [order 1] : [switch_array(i)==0]
  data: switch_array input; delay_array input; outMsg output; inMsg input; i local

== stateflow chart orion_casestudy_8/DelaySwitch24 ==
  state Operation
  state Sending
  (default) -> Operation : {i=0;}
  (junction 7) -> Operation [order 2]
  Sending -> Operation : after(delay_array(i),msec)
      | {receive(inMsg);outMsg.data=0;send(outMsg);}
  Operation -> (junction 7) : inMsg{i = i + 1;}
  (junction 7) -> Sending [order 1] : [switch_array(i)==0]
  data: switch_array input; delay_array input; outMsg output; inMsg input; i local

== stateflow chart orion_casestudy_8/DelaySwitch25 ==
  state Operation
  state Sending
  (default) -> Operation : {i=0;}
  (junction 7) -> Operation [order 2]
  Sending -> Operation : after(delay_array(i),msec)
      | {receive(inMsg);outMsg.data=0;send(outMsg);}
  Operation -> (junction 7) : inMsg{i = i + 1;}
  (junction 7) -> Sending [order 1] : [switch_array(i)==0]
  data: switch_array input; delay_array input; outMsg output; inMsg input; i local

== stateflow chart orion_casestudy_8/DelaySwitch1 ==
  state Operation
  state Sending
  (default) -> Operation : {i=0;}
  (junction 7) -> Operation [order 2]
  Sending -> Operation : after(delay_array(i),msec)
      | {receive(inMsg);outMsg.data=0;send(outMsg);}
  Operation -> (junction 7) : inMsg{i = i + 1;}
  (junction 7) -> Sending [order 1] : [switch_array(i)==0]
  data: switch_array input; delay_array input; outMsg output; inMsg input; i local
